simulink model "CarrotandAdaptive"  (R2020b)
settings: Solver=FixedStepAuto  StartTime=0.0  StopTime=200  FixedStep=0.001  RelTol=1e-3
settings Model: Creator=chainplain  LastModifiedBy=chainplain

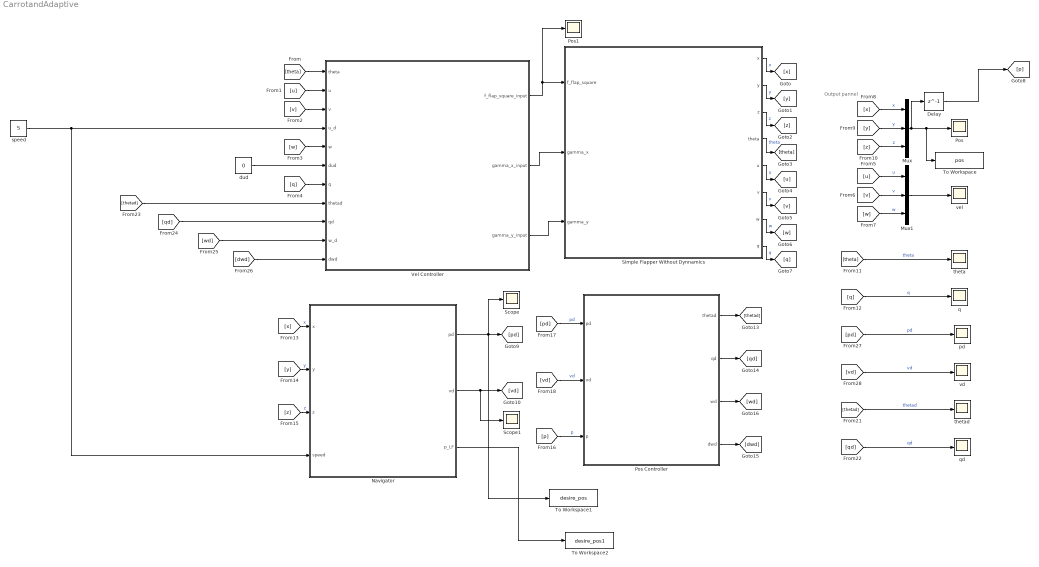
== system CarrotandAdaptive ==
  note: Output pannel
  Delay : Delay  DelayLength=1  InitialCondition=[0;0;0]
  Mux : Mux  Inputs=3
  Mux1 : Mux  Inputs=3
  Navigator : Subsystem  mask{filename=YJF.mat, d_LF=2, d_d=0.5, K_pd1=1.5, K_pd2=1.5, K_pd3=1.5, k_pd=2, K_vd1=1, K_vd2=1, K_vd3=1, xd=0, yd=0, zd=-36.0, vxd=0, vyd=0, vzd=0}
      mask prompts: filename "Trajectory file"; d_LF "nominal distance d_LF"; d_d "denominator d_d"
      mask init:
      | filename_value=get_param(gcb,'filename');
      | load(filename_value);
      | input_P = ['[']
      | for i = 1 : size(P,1) 
      |     input_P = [input_P, num2str(P(i, 1)),','];
      |     input_P = [input_P, num2str(P(i, 2)),','];
      |     input_P = [input_P, num2str(P(i, 3)),';'];
      | end
      | input_P(end) = ']';
      | 
      | set_param([gcb,'/Traj'],'value',input_P)
      | 
      | d_LF_value=get_param(gcb,'d_LF');
      | set_param([gcb,'/d_LF'],'value',d_LF_value);
      | 
      | d_d_value=get_param(gcb,'d_d');
      | set_param([gcb,'/d_d'],'value',d_d_value);
      | 
      | k_pd_value=get_param(gcb,'k_pd');
      | set_param([gcb,'/k_pd'],'gain',k_pd_value);
      | 
      | K_pd1_value=get_param(gcb,'K_pd1');
      | K_pd2_value=get_param(gcb,'K_pd2');
      | K_pd3_value=get_param(gcb,'K_pd3');
      | set_param([gcb,'/K_pd'],'value',['diag([',K_pd1_value,',',...
      |     K_pd2_value,',',K_pd3_value,'])']);
      | 
      | K_vd1_value=get_param(gcb,'K_vd1');
      | K_vd2_value=get_param(gcb,'K_vd2');
      | K_vd3_value=get_param(gcb,'K_vd3');
      | set_param([gcb,'/K_vd'],'value',['diag([',K_vd1_value,',',...
      |     K_vd2_value,',',K_vd3_value,'])']);
      | 
      | xd_value=get_param(gcb,'xd');
      | yd_value=get_param(gcb,'yd');
      | zd_value=get_param(gcb,'zd');
      | set_param([gcb,'/pd_integrator'],'InitialCondition',['[',xd_value,',',...
      |     yd_value,',',zd_value,']']);
      | 
      | vxd_value=get_param(gcb,'vxd');
      | vyd_value=get_param(gcb,'vyd');
      | vzd_value=get_param(gcb,'vzd');
      | set_param([gcb,'/vd_integrator'],'InitialCondition',['[',vxd_value,',',...
      |     vyd_value,',',vzd_value,']']);
      mask DialogControl DescGroupVar Prompt: Nav Paras
      mask DialogControl DescTextVar Prompt: This navigator can be seen as a combination of vector field and carrot chasing. Written by Chainplain.
      mask DialogControl Container7 Prompt: Follow Paras
      mask DialogControl Container3 Prompt: Look forward
      mask DialogControl Container8 Prompt: Filter Paras
      mask DialogControl Container9 Prompt: pos. K_pd=diag([K_pd1,K_pd2,K_pd3])
      mask DialogControl Container11 Prompt: proportional for pos
      mask DialogControl Container10 Prompt: vel. K_vd=diag([K_vd1,K_vd2,K_vd3])
      mask DialogControl Container13 Prompt: Filter Init
      mask DialogControl Container14 Prompt: Filter pos. initial condition
      mask DialogControl Container15 Prompt: Filter vel.  initial condition
      mask Display: image('nav.JPG'); % Use "Edit Image" on toolstrip to change.
  Pos : Scope
  Pos Controller : Subsystem  mask{k_x=5, k_y=5, k_z=1.600, b_z=2}
      mask init:
      | k_x_value=get_param(gcb,'k_x');
      | set_param([gcb,'/kx'],'value',k_x_value);
      | 
      | k_y_value=get_param(gcb,'k_y');
      | set_param([gcb,'/ky'],'value',k_y_value);
      | 
      | k_z_value=get_param(gcb,'k_z');
      | set_param([gcb,'/kz'],'value',k_z_value);
      | 
      | b_z_value=get_param(gcb,'b_z');
      | set_param([gcb,'/bz'],'value',b_z_value);
      mask DialogControl DescGroupVar Prompt: Pos Control Paras
      mask DialogControl DescTextVar Prompt: A simple pos controller. Written by Chainplain.
      mask DialogControl ParameterGroupVar Prompt: positional coefficient
      mask Display: image('pos.JPG'); % Use "Edit Image" on toolstrip to change.
  Pos1 : Scope
  Scope : Scope
  Scope1 : Scope
  Simple Flapper Without Dynnamics : Subsystem  mask{k_T=0.9, k_d0=0.1, k_d1=0.2, k_l0=0.2, k_l1=1, k_d_v=0.3, k_d_w=0.7, g=9.8, X=0, Y=0, Z=-36.0, theta=3.203, u=0.0, v=0, w=0.0}
      mask prompts: k_T "Thurst coefficient:"; k_d0 "Drag coefficient 0:"; k_d1 "Drag coefficient 1:"; k_l0 "Lift coefficient 0:"; k_l1 "Lift coefficient 1:"; k_d_v "Side drag coefficient:"; k_d_w "vertical drag coefficient:"; g "Gravity: (m/s^2)"; X "X(m)"; Y "Y(m)"; Z "Z(m)"; u "u(m/s)"; v "v(m/s)"; w "w(m/s)"
      mask init:
      | k_T_value=get_param(gcb,'k_T');
      | set_param([gcb,'/k_T'],'value',k_T_value);
      | 
      | k_d0_value=get_param(gcb,'k_d0');
      | set_param([gcb,'/k_d0'],'value',k_d0_value);
      | 
      | k_d1_value=get_param(gcb,'k_d1');
      | set_param([gcb,'/k_d1'],'value',k_d1_value);
      | 
      | k_l0_value=get_param(gcb,'k_l0');
      | set_param([gcb,'/k_l0'],'value',k_l0_value);
      | 
      | k_l1_value=get_param(gcb,'k_l1');
      | set_param([gcb,'/k_l1'],'value',k_l1_value);
      | 
      | k_d_v_value=get_param(gcb,'k_d_v');
      | set_param([gcb,'/k_d_v'],'value',k_d_v_value);
      | 
      | k_d_w_value=get_param(gcb,'k_d_w');
      | set_param([gcb,'/k_d_w'],'value',k_d_w_value);
      | 
      | g_value=get_param(gcb,'g');
      | set_param([gcb,'/g'],'value',g_value);
      | 
      | X_value=get_param(gcb,'X');
      | set_param([gcb,'/X_integrator'],'InitialCondition',X_value);
      | 
      | Y_value=get_param(gcb,'Y');
      | set_param([gcb,'/Y_integrator'],'InitialCondition',Y_value);
      | 
      | Z_value=get_param(gcb,'Z');
      | set_param([gcb,'/Z_integrator'],'InitialCondition',Z_value);
      | 
      | theta_value=get_param(gcb,'theta');
      | set_param([gcb,'/theta_integrator'],'InitialCondition',theta_value);
      | 
      | u_value=get_param(gcb,'u');
      | set_param([gcb,'/u_integrator'],'InitialCondition',u_value);
      | 
      | v_value=get_param(gcb,'v');
      | set_param([gcb,'/v_integrator'],'InitialCondition',v_value);
      | 
      | w_value=get_param(gcb,'w');
      | set_param([gcb,'/w_integrator'],'InitialCondition',w_value);
      mask DialogControl DescGroupVar Prompt: Flapper paras
      mask DialogControl DescTextVar Prompt: This is a model of flapping wing vehicle kinematics. Written by Chainplain.
      mask DialogControl Container7 Prompt: System Parameters
      mask DialogControl Container9 Prompt: Initial Conditions
      mask DialogControl Container4 Prompt: Position
      mask DialogControl Container10 Prompt: Heading
      mask DialogControl Container5 Prompt: Velocity in vertical frame
      mask Display: image('$imagefile'); % Use "Edit Image" on toolstrip to change.
  To Workspace : ToWorkspace  VariableName=pos  SaveFormat=Timeseries  SampleTime=-1
  To Workspace1 : ToWorkspace  VariableName=desire_pos  SaveFormat=Timeseries  SampleTime=-1
  To Workspace2 : ToWorkspace  VariableName=desire_pos1  SaveFormat=Timeseries  SampleTime=-1
  Vel Controller : Subsystem  mask{k_u=10, k_w=10, k_theta=2, b_T=0.016, b_d_0=0.0070, b_d_1=0.0070, b_l_0=0.0070, b_l_1=0.013, k_flap_kesi=1, k_x_kesi=1.804, k_y_kesi=0.399, flap_square_max=7.360, flap_square_min=3.250, gammax_max=0.444, gammax_min=-0.420, gammay_max=0.414, gammay_min=-0.444}
      mask prompts: k_u "u (Frame-V X vel.) coefficient"; k_w "w (Frame-V X vel.) coefficient"; k_theta "\theta Heading coefficient"; b_T "hat_k_t update rate"; b_d_0 "hat_k_d_0 update rate"; b_d_1 "hat_k_d_1 update rate"; b_l_0 "hat_k_l_0 update rate"; b_l_1 "hat_k_l_1 update rate"; k_flap_kesi "kesi_flap_damping"; k_x_kesi "kesi_gamma_x_damping"; k_y_kesi "kesi_gamma_y_damping"; flap_square_max "max"; flap_square_min "min"; gammax_max "max"; gammax_min "min"; gammay_max "max"; gammay_min "min"
      mask init:
      | k_u_value=get_param(gcb,'k_u');
      | set_param([gcb,'/k_u'],'value',k_u_value);
      | 
      | k_w_value=get_param(gcb,'k_w');
      | set_param([gcb,'/k_w'],'value',k_w_value);
      | 
      | k_theta_value=get_param(gcb,'k_theta');
      | set_param([gcb,'/k_theta'],'value',k_theta_value);
      | 
      | b_T_value=get_param(gcb,'b_T');
      | set_param([gcb,'/b_T'],'value',b_T_value);
      | 
      | b_d_0_value=get_param(gcb,'b_d_0');
      | set_param([gcb,'/b_d_0'],'value',b_d_0_value);
      | 
      | b_d_1_value=get_param(gcb,'b_d_1');
      | set_param([gcb,'/b_d_1'],'value',b_d_1_value);
      | 
      | b_l_0_value=get_param(gcb,'b_l_0');
      | set_param([gcb,'/b_l_0'],'value',b_l_0_value);
      | 
      | b_l_1_value=get_param(gcb,'b_l_1');
      | set_param([gcb,'/b_l_1'],'value',b_l_1_value);
      | 
      | k_flap_kesi_value=get_param(gcb,'k_flap_kesi');
      | set_param([gcb,'/k_flap_kesi'],'value',k_flap_kesi_value);
      | 
      | k_x_kesi_value=get_param(gcb,'k_x_kesi');
      | set_param([gcb,'/k_x_kesi'],'value',k_x_kesi_value);
      | 
      | k_y_kesi_value=get_param(gcb,'k_y_kesi');
      | set_param([gcb,'/k_y_kesi'],'value',k_y_kesi_value);
      | 
      | f_max_value=get_param(gcb,'flap_square_max');
      | set_param([gcb,'/f_flap_square_sat'],'UpperLimit',f_max_value);
      | f_min_value=get_param(gcb,'flap_square_min');
      | set_param([gcb,'/f_flap_square_sat'],'LowerLimit',f_min_value);
      | 
      | gammax_max_value=get_param(gcb,'gammax_max');
      | set_param([gcb,'/gamma_x_sat'],'UpperLimit',gammax_max_value);
      | gammax_min_value=get_param(gcb,'gammax_min');
      | set_param([gcb,'/gamma_x_sat'],'LowerLimit',gammax_min_value);
      | 
      | gammay_max_value=get_param(gcb,'gammay_max');
      | set_param([gcb,'/gamma_y_sat'],'UpperLimit',gammay_max_value);
      | gammay_min_value=get_param(gcb,'gammay_min');
      | set_param([gcb,'/gamma_y_sat'],'LowerLimit',gammay_min_value);
      mask DialogControl DescGroupVar Prompt: Velocity Controller Paras
      mask DialogControl DescTextVar Prompt: This is an adaptive velocity controller. Written by Chainplain.
      mask DialogControl Container10 Prompt: Feedback
      mask DialogControl Container12 Prompt: Adaptive
      mask DialogControl Container14 Prompt: Saturation
      mask DialogControl Container7 Prompt: Dampings
      mask DialogControl Container8 Prompt: Limits
      mask DialogControl Container9 Prompt: Limits of flap frequency square
      mask DialogControl Container9_copy Prompt: Limits of gammax (pitch)
      mask DialogControl Container9_copy_copy Prompt: Limits of gammay (row)
      mask Display: image('vel.JPG'); % Use "Edit Image" on toolstrip to change.
  dud : Constant  Value=0
  pd : Scope
  q : Scope
  qd : Scope
  speed : Constant  Value=5
  theta : Scope
  thetad : Scope
  vd : Scope
  vel : Scope
  wires:
  speed/1 -> Navigator/4(speed), Vel Controller/4(u_d)
  dud/1 -> Vel Controller/6(dud)
  [thetad] -> Vel Controller/8(thetad)
  [qd] -> Vel Controller/9(qd)
  [wd] -> Vel Controller/10(w_d)
  [dwd] -> Vel Controller/11(dwd)
  Vel Controller/1(f_flap_square_input) -> Pos1/1, Simple Flapper Without Dynnamics/1(f_flap_square)
  Vel Controller/2(gamma_x_input) -> Simple Flapper Without Dynnamics/2(gamma_x)
  Vel Controller/3(gamma_y_input) -> Simple Flapper Without Dynnamics/3(gamma_y)
  Simple Flapper Without Dynnamics/1(x) -> [x]  "x"
  Simple Flapper Without Dynnamics/2(y) -> [y]  "y"
  Simple Flapper Without Dynnamics/3(z) -> [z]  "z"
  Simple Flapper Without Dynnamics/4(theta) -> [theta]  "theta"
  Simple Flapper Without Dynnamics/5(u) -> [u]  "u"
  Simple Flapper Without Dynnamics/6(v) -> [v]  "v"
  Simple Flapper Without Dynnamics/7(w) -> [w]  "w"
  Simple Flapper Without Dynnamics/8(q) -> [q]  "q"
  [theta] -> Vel Controller/1(theta)
  [u] -> Vel Controller/2(u)
  [v] -> Vel Controller/3(v)
  [w] -> Vel Controller/5(w)
  [q] -> Vel Controller/7(q)
  [theta] -> theta/1  "theta"
  [q] -> q/1  "q"
  [v] -> Mux1/2  "v"
  [w] -> Mux1/3  "w"
  [y] -> Mux/2  "y"
  [u] -> Mux1/1  "u"
  Mux1/1 -> vel/1
  [z] -> Mux/3  "z"
  [x] -> Mux/1  "x"
  Mux/1 -> To Workspace/1, Pos/1, Delay/1
  [x] -> Navigator/1(x)  "x"
  [y] -> Navigator/2(y)  "y"
  [z] -> Navigator/3(z)  "z"
  Navigator/1(pd) -> Scope/1, To Workspace1/1, [pd]
  [pd] -> Pos Controller/1(pd)  "pd"
  [vd] -> Pos Controller/2(vd)  "vd"
  [p] -> Pos Controller/3(p)  "p"
  Pos Controller/1(thetad) -> [thetad]
  Pos Controller/2(qd) -> [qd]
  Pos Controller/3(wd) -> [wd]
  Pos Controller/4(dwd) -> [dwd]
  [pd] -> pd/1  "pd"
  [vd] -> vd/1  "vd"
  [thetad] -> thetad/1  "thetad"
  Delay/1 -> [p]
  [qd] -> qd/1  "qd"
  Navigator/3(p_LF) -> To Workspace2/1
  Navigator/2(vd) -> Scope1/1, [vd]

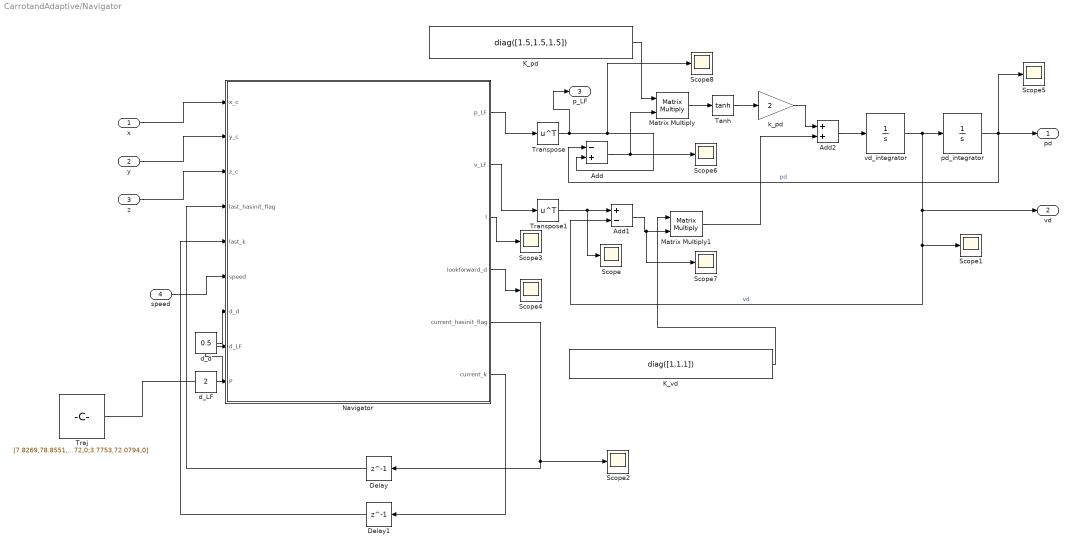
== system CarrotandAdaptive/Navigator ==
  x : Inport
  y : Inport  Port=2
  z : Inport  Port=3
  speed : Inport  Port=4
  Add : Sum  Inputs=-+
  Add1 : Sum  Inputs=+-
  Add2 : Sum
  Delay : Delay  DelayLength=1  InitialCondition=0
  Delay1 : Delay  DelayLength=1  InitialCondition=1
  K_pd : Constant  Value=diag([1.5,1.5,1.5])  VectorParams1D=off
  K_vd : Constant  Value=diag([1,1,1])
  Matrix Multiply : Product  Multiplication=Matrix(*)
  Matrix Multiply1 : Product  Multiplication=Matrix(*)
  Navigator : MATLAB Function  TreatAsAtomicUnit=on
  Scope{,1..8} (9 alike) : Scope
  Tanh : Trigonometry  Operator=tanh
  Traj : Constant  Value=[7.8269,78.8551,0;18.8766,58.0607,0;19.7974,23.2477,0;22.3757,23.014,0;21.639,58.2944,0;31.2155,77.4533,0;48.5267,79.0888,0;49.6317,43.3411,0;48.5267,19.743,0;33.7937,20.4439,0;28.8214,34.6963,0;27.3481,28.1542,0;30.2947,16.472,0;45.9484,15.0701,0;53.4991,16.7056,0;53.4991,78.8551,0;86.4641,80.0234,0;87.2007,73.2477,0;67.1271,72.3131,0;65.1013,52.4533,0;83.1492,52.9206,0;87.0166,49.6495,0;64.9171,46.1449,0;64.733,14.6028,0;7.8269,10.3972,0;3.7753,72.0794,0]
  Transpose : Math  Operator=transpose  SaturateOnIntegerOverflow=on
  Transpose1 : Math  Operator=transpose  SaturateOnIntegerOverflow=on
  d_LF : Constant  Value=2
  d_d : Constant  Value=0.5
  k_pd : Gain  Gain=2
  pd_integrator : Integrator  InitialCondition=[0,0,-36.0]
  vd_integrator : Integrator  InitialCondition=[0,0,0]
  pd : Outport
  vd : Outport  Port=2
  p_LF : Outport  Port=3
  wires:
  Transpose1/1 -> Scope/1, Add1/1
  vd_integrator/1 -> vd/1, Scope1/1, Add1/2, pd_integrator/1  "vd"
  Add/1 -> Scope6/1, Matrix Multiply/2
  Tanh/1 -> k_pd/1
  Navigator/6(current_k) -> Delay1/1
  Add1/1 -> Scope7/1, Matrix Multiply1/2
  k_pd/1 -> Add2/1
  Navigator/2(v_LF) -> Transpose1/1
  K_pd/1 -> Matrix Multiply/1
  pd_integrator/1 -> Scope5/1, pd/1, Add/1  "pd"
  y/1 -> Navigator/2(y_c)
  Navigator/5(current_hasinit_flag) -> Scope2/1, Delay/1
  d_d/1 -> Navigator/7(d_d)
  Matrix Multiply/1 -> Tanh/1
  d_LF/1 -> Navigator/8(d_LF)
  Transpose/1 -> p_LF/1, Scope8/1, Add/2
  Matrix Multiply1/1 -> Add2/2
  Delay1/1 -> Navigator/5(last_k)
  z/1 -> Navigator/3(z_c)
  speed/1 -> Navigator/6(speed)
  Navigator/1(p_LF) -> Transpose/1
  Add2/1 -> vd_integrator/1
  Delay/1 -> Navigator/4(last_hasinit_flag)
  K_vd/1 -> Matrix Multiply1/1
  x/1 -> Navigator/1(x_c)
  Traj/1 -> Navigator/9(P)
  Navigator/3(l) -> Scope3/1
  Navigator/4(lookforward_d) -> Scope4/1

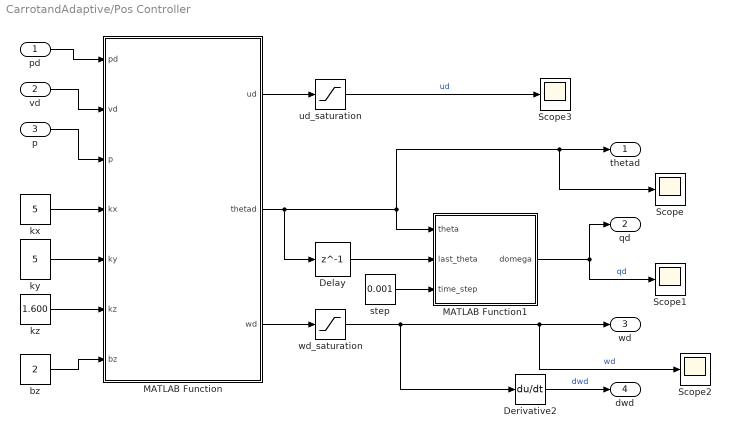
== system CarrotandAdaptive/Pos Controller ==
  pd : Inport
  vd : Inport  Port=2
  p : Inport  Port=3
  Delay : Delay  DelayLength=1  InitialCondition=0
  Derivative2 : Derivative  CoefficientInTFapproximation=10
  MATLAB Function : MATLAB Function  TreatAsAtomicUnit=on
  MATLAB Function1 : MATLAB Function  TreatAsAtomicUnit=on
  Scope{,1..3} (4 alike) : Scope
  bz : Constant  Value=2
  kx : Constant  Value=5
  ky : Constant  Value=5
  kz : Constant  Value=1.600
  step : Constant  Value=0.001
  ud_saturation : Saturate  UpperLimit=7  LowerLimit=4.5
  wd_saturation : Saturate  UpperLimit=2  LowerLimit=-2
  thetad : Outport
  qd : Outport  Port=2
  wd : Outport  Port=3
  dwd : Outport  Port=4
  wires:
  MATLAB Function/3(wd) -> wd_saturation/1
  ud_saturation/1 -> Scope3/1  "ud"
  MATLAB Function/2(thetad) -> Delay/1, MATLAB Function1/1(theta), Scope/1, thetad/1
  vd/1 -> MATLAB Function/2(vd)
  kx/1 -> MATLAB Function/4(kx)
  ky/1 -> MATLAB Function/5(ky)
  p/1 -> MATLAB Function/3(p)
  wd_saturation/1 -> Scope2/1, wd/1, Derivative2/1  "wd"
  MATLAB Function/1(ud) -> ud_saturation/1
  kz/1 -> MATLAB Function/6(kz)
  pd/1 -> MATLAB Function/1(pd)
  Derivative2/1 -> dwd/1  "dwd"
  MATLAB Function1/1(domega) -> Scope1/1, qd/1  "qd"
  step/1 -> MATLAB Function1/3(time_step)
  Delay/1 -> MATLAB Function1/2(last_theta)
  bz/1 -> MATLAB Function/7(bz)

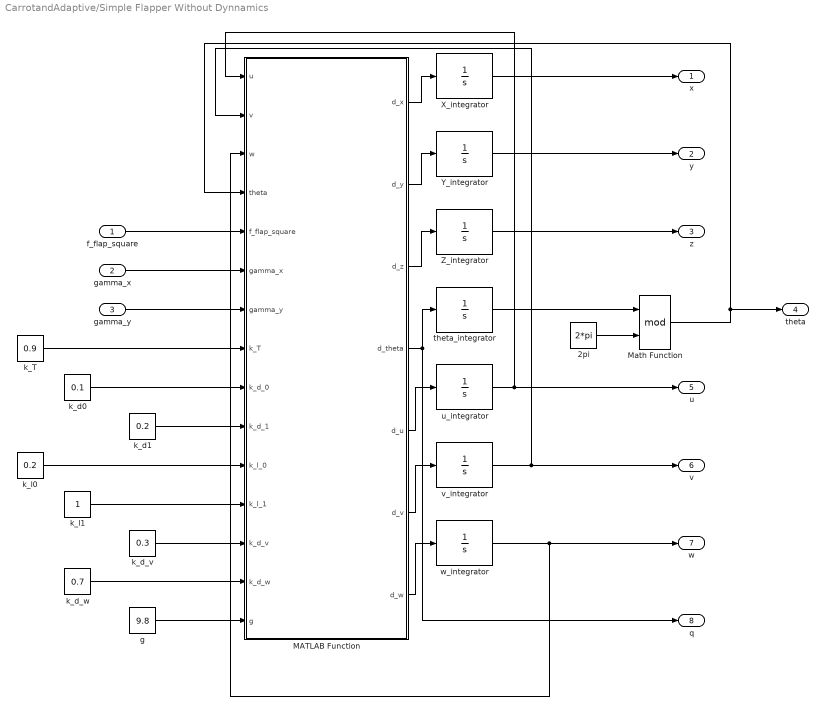
== system CarrotandAdaptive/Simple Flapper Without Dynnamics ==
  f_flap_square : Inport
  gamma_x : Inport  Port=2
  gamma_y : Inport  Port=3
  2pi : Constant  Value=2*pi
  MATLAB Function : MATLAB Function  TreatAsAtomicUnit=on
  Math Function : Math  Operator=mod  SaturateOnIntegerOverflow=on
  X_integrator : Integrator
  Y_integrator : Integrator
  Z_integrator : Integrator  InitialCondition=-36.0
  g : Constant  Value=9.8
  k_T : Constant  Value=0.9
  k_d0 : Constant  Value=0.1
  k_d1 : Constant  Value=0.2
  k_d_v : Constant  Value=0.3
  k_d_w : Constant  Value=0.7
  k_l0 : Constant  Value=0.2
  k_l1 : Constant
  theta_integrator : Integrator  InitialCondition=3.203
  u_integrator : Integrator  InitialCondition=0.0
  v_integrator : Integrator
  w_integrator : Integrator  InitialCondition=0.0
  x : Outport
  y : Outport  Port=2
  z : Outport  Port=3
  theta : Outport  Port=4
  u : Outport  Port=5
  v : Outport  Port=6
  w : Outport  Port=7
  q : Outport  Port=8
  wires:
  MATLAB Function/1(d_x) -> X_integrator/1
  MATLAB Function/4(d_theta) -> theta_integrator/1, q/1
  g/1 -> MATLAB Function/15(g)
  u_integrator/1 -> u/1, MATLAB Function/1(u)
  k_T/1 -> MATLAB Function/8(k_T)
  v_integrator/1 -> v/1, MATLAB Function/2(v)
  MATLAB Function/6(d_v) -> v_integrator/1
  gamma_x/1 -> MATLAB Function/6(gamma_x)
  MATLAB Function/7(d_w) -> w_integrator/1
  Math Function/1 -> theta/1, MATLAB Function/4(theta)
  Z_integrator/1 -> z/1
  MATLAB Function/5(d_u) -> u_integrator/1
  w_integrator/1 -> w/1, MATLAB Function/3(w)
  X_integrator/1 -> x/1
  Y_integrator/1 -> y/1
  f_flap_square/1 -> MATLAB Function/5(f_flap_square)
  MATLAB Function/3(d_z) -> Z_integrator/1
  k_l1/1 -> MATLAB Function/12(k_l_1)
  k_l0/1 -> MATLAB Function/11(k_l_0)
  MATLAB Function/2(d_y) -> Y_integrator/1
  k_d0/1 -> MATLAB Function/9(k_d_0)
  k_d1/1 -> MATLAB Function/10(k_d_1)
  gamma_y/1 -> MATLAB Function/7(gamma_y)
  theta_integrator/1 -> Math Function/1
  2pi/1 -> Math Function/2
  k_d_v/1 -> MATLAB Function/13(k_d_v)
  k_d_w/1 -> MATLAB Function/14(k_d_w)

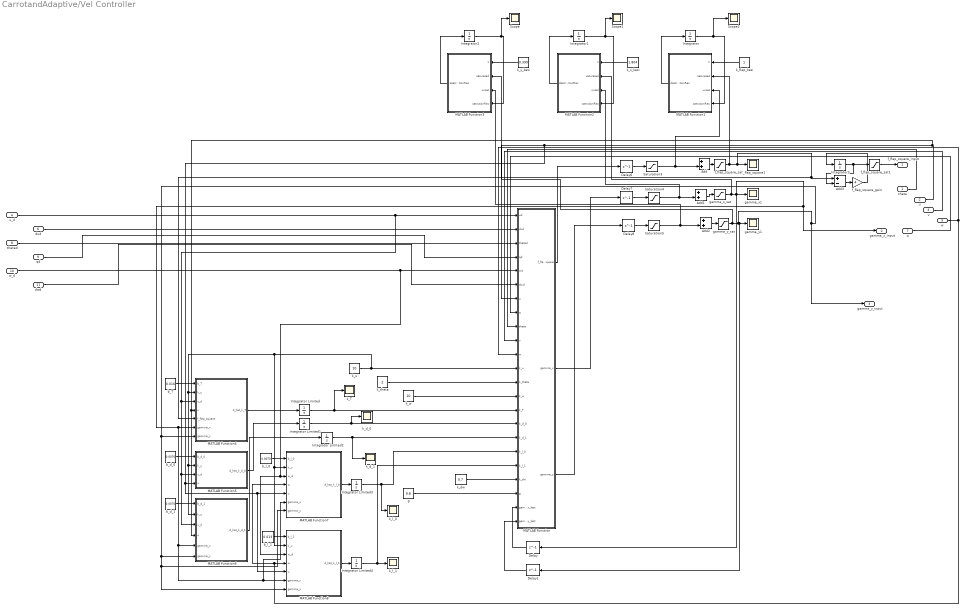
== system CarrotandAdaptive/Vel Controller ==
  theta : Inport
  u : Inport  Port=2
  v : Inport  Port=3
  u_d : Inport  Port=4
  w : Inport  Port=5
  dud : Inport  Port=6
  q : Inport  Port=7
  thetad : Inport  Port=8
  qd : Inport  Port=9
  w_d : Inport  Port=10
  dwd : Inport  Port=11
  Add : Sum
  Add1 : Sum
  Add2 : Sum
  Add3 : Sum  Inputs=+-
  Delay{,1,7..8} (4 alike) : Delay  DelayLength=1  InitialCondition=0
  Delay6 : Delay  DelayLength=1  InitialCondition=5
  Integrator{,1..3} (4 alike) : Integrator
  Integrator Limited : Integrator  InitialCondition=0.5  LimitOutput=on  UpperSaturationLimit=1.5  LowerSaturationLimit=0.5
  Integrator Limited1 : Integrator  LimitOutput=on  UpperSaturationLimit=0.5  LowerSaturationLimit=0
  Integrator Limited2 : Integrator  LimitOutput=on  UpperSaturationLimit=0.5  LowerSaturationLimit=0
  Integrator Limited3 : Integrator  LimitOutput=on  UpperSaturationLimit=0.5  LowerSaturationLimit=0
  Integrator Limited4 : Integrator  InitialCondition=1  LimitOutput=on  UpperSaturationLimit=1.5  LowerSaturationLimit=0.5
  MATLAB Function : MATLAB Function  TreatAsAtomicUnit=on
  MATLAB Function1 : MATLAB Function  TreatAsAtomicUnit=on
  MATLAB Function2 : MATLAB Function  TreatAsAtomicUnit=on
  MATLAB Function3 : MATLAB Function  TreatAsAtomicUnit=on
  MATLAB Function4 : MATLAB Function  TreatAsAtomicUnit=on
  MATLAB Function5 : MATLAB Function  TreatAsAtomicUnit=on
  MATLAB Function6 : MATLAB Function  TreatAsAtomicUnit=on
  MATLAB Function7 : MATLAB Function  TreatAsAtomicUnit=on
  MATLAB Function8 : MATLAB Function  TreatAsAtomicUnit=on
  Saturation3 : Saturate  UpperLimit=8  LowerLimit=2
  Saturation4 : Saturate  UpperLimit=1  LowerLimit=-1
  Saturation5 : Saturate  UpperLimit=1  LowerLimit=-1
  Scope : Scope
  Scope1 : Scope
  Scope2 : Scope
  b_T : Constant  Value=0.016
  b_d_0 : Constant  Value=0.0070
  b_d_1 : Constant  Value=0.0070
  b_l_0 : Constant  Value=0.0070
  b_l_1 : Constant  Value=0.013
  f_flap_square1 : Scope
  f_flap_square_gain : Gain  Gain=4
  f_flap_square_sat : Saturate  UpperLimit=7.360  LowerLimit=3.250
  f_flap_square_sat1 : Saturate  UpperLimit=7.360  LowerLimit=3.250
  g : Constant  Value=9.8
  gamma_x1 : Scope
  gamma_x_sat : Saturate  UpperLimit=0.444  LowerLimit=-0.420
  gamma_y1 : Scope
  gamma_y_sat : Saturate  UpperLimit=0.414  LowerLimit=-0.444
  k_T : Scope
  k_d_0 : Scope
  k_d_1 : Scope
  k_dw : Constant  Value=0.7
  k_flap_kesi : Constant
  k_l_0 : Scope
  k_l_1 : Scope
  k_theta : Constant  Value=2
  k_u : Constant  Value=10
  k_w : Constant  Value=10
  k_x_kesi : Constant  Value=1.804
  k_y_kesi : Constant  Value=0.399
  f_flap_square_input : Outport
  gamma_x_input : Outport  Port=2
  gamma_y_input : Outport  Port=3
  wires:
  MATLAB Function/3(gamma_y) -> Delay8/1
  u_d/1 -> MATLAB Function4/3(u_d), MATLAB Function6/3(u_d), MATLAB Function5/3(u_d), MATLAB Function/1(ud)
  Saturation5/1 -> MATLAB Function3/3(unsat), Add2/2
  k_w/1 -> MATLAB Function/14(k_w)
  Integrator1/1 -> Scope1/1, MATLAB Function2/4(satrutionRec)
  f_flap_square_sat/1 -> MATLAB Function1/2(saturated), Add3/1, MATLAB Function4/5(f_flap_square), f_flap_square1/1
  w_d/1 -> MATLAB Function8/3(w_d), MATLAB Function7/3(w_d), MATLAB Function/5(wd)
  theta/1 -> MATLAB Function/9(theta)
  k_theta/1 -> MATLAB Function/13(k_theta)
  k_u/1 -> MATLAB Function8/2(k_u), MATLAB Function7/2(k_u), MATLAB Function6/2(k_u), MATLAB Function5/2(k_u), MATLAB Function4/2(k_u), MATLAB Function/12(k_u)
  Saturation4/1 -> MATLAB Function2/3(unsat), Add1/2
  Integrator Limited4/1 -> k_l_1/1, MATLAB Function/19(k_l_1)
  b_l_0/1 -> MATLAB Function7/1(b_l_0)
  b_l_1/1 -> MATLAB Function8/1(b_l_1)
  MATLAB Function4/1(d_hat_k_T) -> Integrator Limited/1
  k_dw/1 -> MATLAB Function/20(k_dw)
  Integrator Limited2/1 -> k_d_1/1, MATLAB Function/17(k_d_1)
  MATLAB Function/2(gamma_x) -> Delay7/1
  Integrator Limited3/1 -> k_l_0/1, MATLAB Function/18(k_l_0)
  Integrator Limited/1 -> k_T/1, MATLAB Function/15(k_T)
  Delay7/1 -> Saturation4/1
  Integrator Limited1/1 -> k_d_0/1, MATLAB Function/16(k_d_0)
  MATLAB Function/1(f_flap_square) -> Delay6/1
  Delay6/1 -> Saturation3/1
  dud/1 -> MATLAB Function/2(dud)
  Integrator/1 -> Scope2/1, MATLAB Function1/4(satrutionRec)
  w/1 -> MATLAB Function/11(w), MATLAB Function7/4(w), MATLAB Function8/4(w)
  MATLAB Function2/1(dsatrutionRec) -> Integrator1/1
  k_x_kesi/1 -> MATLAB Function2/1(k)
  MATLAB Function3/1(dsatrutionRec) -> Integrator2/1
  qd/1 -> MATLAB Function/4(qd)
  q/1 -> MATLAB Function/8(q)
  b_d_0/1 -> MATLAB Function5/1(b_d_0)
  Delay/1 -> MATLAB Function/22(gamma_x_last)
  Delay1/1 -> MATLAB Function/23(gamma_y_last)
  b_d_1/1 -> MATLAB Function6/1(b_d_1)
  Delay8/1 -> Saturation5/1
  k_y_kesi/1 -> MATLAB Function3/1(k)
  g/1 -> MATLAB Function/21(g)
  Add/1 -> f_flap_square_sat/1
  v/1 -> MATLAB Function/10(v)
  Add1/1 -> gamma_x_sat/1
  Add2/1 -> gamma_y_sat/1
  b_T/1 -> MATLAB Function4/1(b_T)
  Saturation3/1 -> MATLAB Function1/3(unsat), Add/2
  k_flap_kesi/1 -> MATLAB Function1/1(k)
  MATLAB Function1/1(dsatrutionRec) -> Integrator/1
  Integrator2/1 -> Scope/1, MATLAB Function3/4(satrutionRec)
  u/1 -> MATLAB Function6/4(u), MATLAB Function4/4(u), MATLAB Function8/5(u), MATLAB Function7/5(u), MATLAB Function5/4(u), MATLAB Function/7(u)
  MATLAB Function5/1(d_hat_k_d_0) -> Integrator Limited1/1
  MATLAB Function6/1(d_hat_k_d_1) -> Integrator Limited2/1
  MATLAB Function8/1(d_hat_k_l_1) -> Integrator Limited4/1
  MATLAB Function7/1(d_hat_k_l_0) -> Integrator Limited3/1
  thetad/1 -> MATLAB Function/3(thetad)
  dwd/1 -> MATLAB Function/6(dwd)
  Integrator3/1 -> f_flap_square_sat1/1, Add3/2
  Add3/1 -> f_flap_square_gain/1
  f_flap_square_gain/1 -> Integrator3/1
  gamma_x_sat/1 -> MATLAB Function2/2(saturated), Delay/1, gamma_x_input/1, MATLAB Function7/6(gamma_x), MATLAB Function8/6(gamma_x), MATLAB Function6/5(gamma_x), MATLAB Function4/6(gamma_x), gamma_x1/1
  gamma_y_sat/1 -> MATLAB Function3/2(saturated), gamma_y_input/1, MATLAB Function8/7(gamma_y), MATLAB Function7/7(gamma_y), MATLAB Function6/6(gamma_y), MATLAB Function4/7(gamma_y), Delay1/1, gamma_y1/1
  f_flap_square_sat1/1 -> f_flap_square_input/1

== matlab function CarrotandAdaptive/Vel Controller/MATLAB Function2 ==
  data: k input; dsatrutionRec output; saturated input; unsat input; satrutionRec input
function dsatrutionRec = CaldsatrutionRec(k, saturated, unsat, satrutionRec)

dsatrutionRec = - k * satrutionRec + unsat - saturated;

== matlab function CarrotandAdaptive/Vel Controller/MATLAB Function3 ==
  data: k input; dsatrutionRec output; saturated input; unsat input; satrutionRec input
function dsatrutionRec = CaldsatrutionRec(k, saturated, unsat, satrutionRec)

dsatrutionRec = - k * satrutionRec + unsat - saturated;

== matlab function CarrotandAdaptive/Vel Controller/MATLAB Function4 ==
  data: b_T input; k_u input; u_d input; u input; d_hat_k_T output; f_flap_square input; gamma_x input; gamma_y input
function d_hat_k_T = para_update(b_T, k_u, u_d, u, f_flap_square, gamma_x, gamma_y)

d_hat_k_T = - b_T / k_u * (u_d - u) * f_flap_square * sqrt(1 - gamma_x^2 - gamma_y^2);

== matlab function CarrotandAdaptive/Vel Controller/MATLAB Function5 ==
  data: b_d_0 input; k_u input; u_d input; u input; d_hat_k_d_0 output
function d_hat_k_d_0 = para_update(b_d_0, k_u, u_d, u)

d_hat_k_d_0 =  b_d_0 / k_u * (u_d - u) * u * u;

== matlab function CarrotandAdaptive/Vel Controller/MATLAB Function6 ==
  data: b_d_1 input; k_u input; u_d input; u input; d_hat_k_d_1 output; gamma_x input; gamma_y input
function d_hat_k_d_1 = para_update(b_d_1, k_u, u_d, u, gamma_x, gamma_y)

d_hat_k_d_1 = b_d_1 / k_u * (u_d - u) * sqrt(1 - gamma_x^2 - gamma_y^2) * u * u;

== matlab function CarrotandAdaptive/Vel Controller/MATLAB Function7 ==
  data: b_l_0 input; k_u input; w_d input; w input; u input; d_hat_k_l_0 output; gamma_x input; gamma_y input
function d_hat_k_l_0 = para_update(b_l_0, k_u, w_d, w, u, gamma_x, gamma_y)

d_hat_k_l_0 = - b_l_0 / k_u * (w_d - w) * u * u * sqrt(1 - gamma_x^2 - gamma_y^2);

== matlab function CarrotandAdaptive/Vel Controller/MATLAB Function8 ==
  data: b_l_1 input; k_u input; w_d input; w input; u input; d_hat_k_l_1 output; gamma_x input; gamma_y input
function d_hat_k_l_1 = para_update(b_l_1, k_u, w_d, w, u, gamma_x, gamma_y)

d_hat_k_l_1 =  b_l_1 / k_u * (w_d - w) * u * u * sqrt(1 - gamma_x^2 - gamma_y^2) * gamma_x;

== matlab function CarrotandAdaptive/Navigator/Navigator ==
  data: x_c input; p_LF output; y_c input; z_c input; v_LF output; l output; lookforward_d output; last_hasinit_flag input; current_hasinit_flag output; last_k input; current_k output; speed input; d_d input; d_LF input; P input
function [p_LF, v_LF, l,lookforward_d, current_hasinit_flag, current_k]= CalcRef(x_c, y_c, z_c, last_hasinit_flag,  last_k, ...
                                                             speed, d_d, d_LF, P)
%% Load the path
points_num = size(P, 1);
%% Check if initial condition
p_c = [x_c, y_c, z_c];
if ~last_hasinit_flag
    P_C = ones(points_num, 1) * p_c;
    Diff = P - P_C;
    Diff_square = Diff(:,1).^2 + Diff(:,2).^2 + Diff(:,3).^2;
    [~,current_k] = min(Diff_square);
else
%     disp(['last_k:',num2str(last_k)]);
    current_k = last_k;
end

current_hasinit_flag = 1;
%% Computation 
p_k = P(current_k, :);
next_k = current_k + 1;
while next_k > points_num
   next_k = next_k - points_num;
end

p_k_plus_1 = P(next_k, :);

l = (p_c - p_k) * (p_k_plus_1 - p_k)' / norm( p_k_plus_1 - p_k )^2;
if l < 0
    l = 0;
end
if l > 1
    l = 1;
end


p_r = l * (p_k_plus_1 - p_k) + p_k;


lookforward_d = d_d * d_LF / ( norm( p_r - p_c) + d_d);


k_LF = current_k;
if k_LF > points_num
   k_LF = k_LF - points_num;
end
next_k_LF = k_LF + 1;
if next_k_LF > points_num
   next_k_LF = next_k_LF - points_num;
end

if norm( P(next_k_LF,:) - p_r) >= lookforward_d
    p_LF = p_r + lookforward_d * ( P(next_k_LF,:) - p_k) / norm(  P(next_k_LF,:) - p_k );
    v_LF = speed * ( P(next_k_LF,:) - p_k) / norm(  P(next_k_LF,:) - p_k );
else
    k_LF = k_LF + 1;
    if k_LF > points_num
       k_LF = k_LF - points_num;
    end
    next_k_LF = k_LF + 1;
    if next_k_LF > points_num
       next_k_LF = next_k_LF - points_num;
    end
    
%     disp(['next_k_LF:',num2str(next_k_LF)]);
    
    lookforward_d = lookforward_d - norm( p_k_plus_1 - p_r);
    while norm( P(next_k_LF, :) - P(k_LF, :)) < lookforward_d       
        lookforward_d = lookforward_d - norm( P(next_k_LF, :) - P(k_LF, :));
            k_LF = k_LF + 1;
            if k_LF > points_num
               k_LF = k_LF - points_num;
            end
            next_k_LF = k_LF + 1;
            if next_k_LF > points_num
               next_k_LF = next_k_LF - points_num;
            end           
    end
%     disp(['k_LF:',num2str(k_LF)]);
    p_LF = P(k_LF, :) + lookforward_d * (P(next_k_LF, :) - P(k_LF, :)) / norm( P(next_k_LF, :) - P(k_LF, :) );
    v_LF = speed * (P(next_k_LF, :) - P(k_LF, :)) / norm( P(next_k_LF, :) - P(k_LF, :) );
end

if  norm(p_c -p_k) > norm(p_k - p_k_plus_1) 
    current_hasinit_flag = 0;
end
    
if  norm(p_c - p_k_plus_1) < d_LF/2
    current_k = next_k;
end


end

== matlab function CarrotandAdaptive/Pos Controller/MATLAB Function ==
  data: pd input; ud output; vd input; p input; thetad output; wd output; kx input; ky input; kz input; bz input
function [ud, thetad, wd] = computeInput(pd, vd, p,  kx, ky, kz, bz)
xd = pd(1);
yd = pd(2);
zd = pd(3);

vdx = vd(1);
vdy = vd(2);
vdz = vd(3);

x = p(1);
y = p(2);
z = p(3);

ud = sqrt ( (vdx  + ky * (yd - y) )^2 ...
          + (vdy  + kx * (xd - x) )^2);
thetad = atan2 (vdy + ky * (yd - y), vdx + kx * (xd - x));
wd = vdz + kz * tanh(bz * zd - bz *z);

== matlab function CarrotandAdaptive/Pos Controller/MATLAB Function1 ==
  data: theta input; domega output; last_theta input; time_step input
function domega = fcn(theta, last_theta,time_step)
mag = sqrt((cos(theta) - cos(last_theta))^2 + (sin(theta) - sin(last_theta))^2 );
d_x = cos(theta) - cos(last_theta);
d_y = sin(theta) - sin(last_theta);
signal_v = sign (cos(theta) * d_y -  sin(last_theta) * d_x);
domega = signal_v * mag / time_step;

== matlab function CarrotandAdaptive/Vel Controller/MATLAB Function ==
  data: ud input; dud input; thetad input; qd input; wd input; dwd input; u input; q input; theta input; v input; w input; k_u input; k_theta input; k_w input; k_T input; f_flap_square output; gamma_x output; k_d_0 input; k_d_1 input; k_l_0 input; k_l_1 input; k_dw input; g input; gamma_y output; gamma_x_last input; gamma_y_last input
function [f_flap_square, gamma_x, gamma_y] =...
    rawCon(ud, dud, thetad, qd, wd, dwd, u, q,theta, v, ...
    w, k_u, k_theta, k_w, k_T, k_d_0, k_d_1, k_l_0,  k_l_1, k_dw,g, gamma_x_last, gamma_y_last)
SMALLCONSTANT = 1e-3;
gamma_z_last =sqrt(1 - gamma_x_last^ 2 - gamma_y_last^ 2) + SMALLCONSTANT;
u_lower_limmit = 1e-3;
if u < u_lower_limmit
   u = u_lower_limmit;
end

gamma_x   = k_l_1^(-1) * gamma_z_last ^ (-1) *  u^(-2)  * ( k_l_0 * u^2 * gamma_z_last- k_dw * abs(w)*w - g) ...
            -k_l_1^(-1) * gamma_z_last ^ (-1) *  u^(-2)*  ( k_w * (wd - w) + dwd);
signplus = sign (sin( thetad - theta));
if signplus == 0
   signplus = 1; 
end
gamma_y   = (k_theta * signplus * abs(sin( (thetad - theta)/2))+ qd);
% gamma_z   = sqrt(1 - gamma_x^2 - gamma_y^2);
f_flap_square = k_T^(-1) * gamma_z_last ^ (-1) * (k_d_0 * u^2 + k_d_1 * gamma_x^2 * gamma_y^2 * u^2 + q * v) +...
             k_T ^ (-1) * gamma_z_last ^ (-1) * ( k_u * (ud - u) + dud);

== matlab function CarrotandAdaptive/Simple Flapper Without Dynnamics/MATLAB Function ==
  data: u input; d_x output; v input; w input; theta input; f_flap_square input; gamma_x input; gamma_y input; k_T input; k_d_0 input; k_d_1 input; k_l_0 input; k_l_1 input; k_d_v input; k_d_w input; g input; d_y output; d_z output; d_theta output; d_u output; d_v output; d_w output
function [d_x, d_y, d_z, d_theta, d_u, d_v, d_w]= Kinemaic(u, v, w, theta, f_flap_square, ...
                gamma_x, gamma_y, k_T, k_d_0, k_d_1, k_l_0,  k_l_1, k_d_v, k_d_w, g)
d_x = u * cos(theta) - v * sin(theta);
d_y = u * sin(theta) + v * cos(theta);
d_z = w;
d_theta = ( k_l_0 * u - k_l_1 * gamma_x * u) * gamma_y;
gamma_z = sqrt(1 - gamma_x^2 - gamma_y^2);
d_u = k_T * f_flap_square * gamma_z- k_d_0 * u ^2 - k_d_1 * ( gamma_x^2 + gamma_y^2 ) * u ^2 - d_theta * v;
d_v = ( k_l_0 * u^2 - k_l_1 * gamma_x * u^2) * gamma_y + d_theta * u - k_d_v * v * abs(v);
d_w = -k_T * f_flap_square * gamma_x + ( k_l_0 * u^2 - k_l_1 * gamma_x * u^2) * sqrt( 1 - gamma_x^2 - gamma_y^2 ) - k_d_w * w * abs(w) - g;

== matlab function CarrotandAdaptive/Vel Controller/MATLAB Function1 ==
  data: k input; dsatrutionRec output; saturated input; unsat input; satrutionRec input
function dsatrutionRec = CaldsatrutionRec(k, saturated, unsat, satrutionRec)

dsatrutionRec = - k * satrutionRec + unsat - saturated;
